simulink model "fmr_ut"  (Simulink 8.1)
settings: Solver=FixedStepDiscrete  StartTime=0.0  StopTime=Inf  FixedStep=0.005  RelTol=1e-3
PostLoadFcn:
  | , if any(exist('dsrtsu_mdlpostloadfcn', 'file') == [2, 3, 6]), try dsrtsu_mdlpostloadfcn('Execute', bdroot); catch fprintf('Error in PostLoadFcn (dsrtsu_mdlpostloadfcn) for model "%s":\n %s\n', bdroot, lasterr); end, end,
libraries: siltestlib x6, fmr x1
settings Model: DSRTSU_INTERNAL_RTI_VER=450  DSRTSU_INTERNAL_RTI_TYPE=rti1401  RTICANMMDATA=struct('GeneralSetupData',struct('modelroot','D:\ELN150201_TAIWAN\trunk\AdasDragon\software\sw_development\arch\app\acc','generalsettings',struct('filesettings',struct('destfolder',struct('Name','RTICANMM_FILES','Check',1),'buildfolder',struct('Name','.','Check',1),'AbsDestfolder',struct('Name','D:\ELN150201_TAIWAN\trunk\AdasDragon\software\sw_development\arch\app\acc\RTICANMM_FILES'),'AbsBuildfolder',struct('Name','D:\ELN150201_TAIWAN\trunk\AdasDragon\software\sw_development\arch\app\acc'))),'options',struct('addpaths',1,'rmpaths',1,'addtrcexclusion',logical(1),'cannavigator',struct('checkmonitoring',0),'show_usrtrc',0,'use_usrtrc',0),'advanced',struct('options',[1 1 1 1 1 1 1 1 1 1 1 1 1 1 1 1 1 1 1 1 1 1 1 1 1 1 1 1 1 1 1 1 1 1 1 1 1 1 1 1 1 1 1 1 1 1 1 1 1 1 1 1 1 1 1 1 1 1 1 1 1 1 1 1 1 1 1 1 1 1 1 1 1 1 1 1 1 1 1 1 1 1 1 1 1 1 1 1 1 1 1 1 1 1 1 1 1 1 1 1]),'MPSetup',{{}},'modelname','fmr_ut','block','fmr_ut'))  DSRTSU_INTERNAL_RTIFPGA=40  Creator=AT015411  LastModifiedBy=AT015555  BufferReuse=off
settings DataIOCC: SignalLoggingSaveFormat=Dataset
settings OptimizationCC: BlockReduction=off  OptimizeBlockIOStorage=off  BufferReuse=off  ExpressionFolding=off  ExpressionDepthLimit=128  LocalBlockOutputs=off
settings DebuggingCC: FcnCallInpInsideContextMsg=EnableAllAsError
settings HardwareCC: ProdIntDivRoundTo=Zero  ProdEndianess=BigEndian  ProdHWDeviceType=Generic->Custom  TargetIntDivRoundTo=Zero  TargetEndianess=BigEndian  TargetHWDeviceType=Generic->Custom
settings RTWCC: SystemTargetFile=rti1005.tlc  MakeCommand=make_rti  TemplateMakefile=rti1005.tmf  Description=dSPACE DS1005 Hardware Platform  ProcessScript=rti1005_make_rtw_hook
settings STFCustomTargetCC: CodeReplacementLibrary=ANSI_C  ParMdlRefBuildCompliant=on  GeneratePreprocessorConditionals=Disable all  MatFileLogging=on  SystemTargetFile=rti1005.tlc
settings GRTTargetCC: CompOptLevelCompliant=off  ConcurrentExecutionCompliant=off  ExtModeMexFile=noextcomm
settings CustomProperty: DataType=RTWOptions_EnumType_C__Program Files (x86)_dSPACE RCPHIL 2014-B_MATLAB_RTI_RTI1401_TLC_rti1005_1InitialSimState  Value=RUN
settings EnumStrPairs: String=RUN

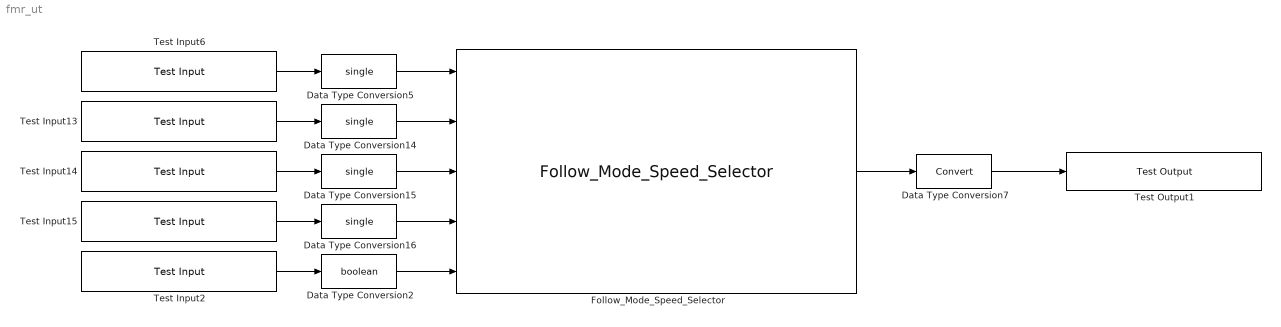
== system fmr_ut ==
  Data Type Conversion{5,14..16} (4 alike) : DataTypeConversion  OutDataTypeStr=single
  Data Type Conversion2 : DataTypeConversion  OutDataTypeStr=boolean
  Data Type Conversion7 : DataTypeConversion
  Follow_Mode_Speed_Selector : fmr/Follow_Mode_Speed_Selector
  Test Input13 : siltestlib/Test Input  varname=VACC_ACCTargetVehSpd_mps  sampletime=0.005
  Test Input14 : siltestlib/Test Input  varname=VIFO_ACCVehClearance:m  sampletime=0.005
  Test Input15 : siltestlib/Test Input  varname=VACC_DesiredDistance_m  sampletime=0.005
  Test Input2 : siltestlib/Test Input  varname=VACC_ACCDistControlSel_flg  sampletime=0.005
  Test Input6 : siltestlib/Test Input  varname=VACC_FollowModeSetSpd_mps  sampletime=0.005
  Test Output1 : siltestlib/Test Output  varname=VACC_MinFollowModelSpd_mps  sampletime=-1
  wires:
  Data Type Conversion7/1 -> Test Output1/1
  Follow_Mode_Speed_Selector/1 -> Data Type Conversion7/1
  Test Input6/1 -> Data Type Conversion5/1
  Data Type Conversion5/1 -> Follow_Mode_Speed_Selector/1
  Test Input2/1 -> Data Type Conversion2/1
  Data Type Conversion2/1 -> Follow_Mode_Speed_Selector/5
  Test Input13/1 -> Data Type Conversion14/1
  Data Type Conversion14/1 -> Follow_Mode_Speed_Selector/2
  Test Input14/1 -> Data Type Conversion15/1
  Data Type Conversion15/1 -> Follow_Mode_Speed_Selector/3
  Test Input15/1 -> Data Type Conversion16/1
  Data Type Conversion16/1 -> Follow_Mode_Speed_Selector/4
